simulink model "indicator_controller"  (R2025a)
settings: Solver=VariableStepAuto  StartTime=0.0  StopTime=10.0  RelTol=1e-3
settings Model: Creator=admin  LastModifiedBy=admin

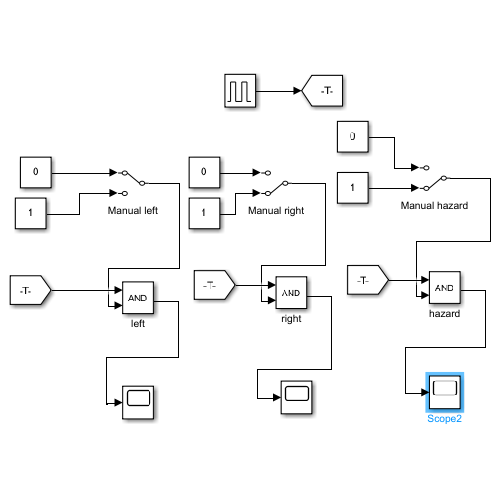
[thumbnail: Simulink's stored preview of the top-level diagram]
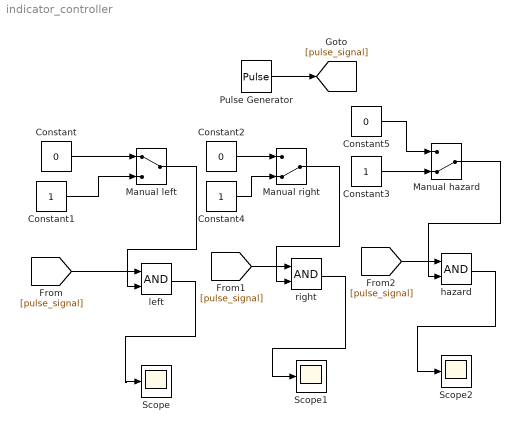
== system indicator_controller ==
  Constant : Constant  Value=0
  Constant1 : Constant
  Constant2 : Constant  Value=0
  Constant3 : Constant
  Constant4 : Constant
  Constant5 : Constant  Value=0
  Manual hazard : ManualSwitch  CurrentSetting=0
  Manual left : ManualSwitch
  Manual right : ManualSwitch  CurrentSetting=0
  Pulse Generator : DiscretePulseGenerator  PulseType=Time based  PulseWidth=50
  Scope : Scope
      settings: ActiveDisplayYMinimum=-1  ActiveDisplayYMaximum=1
  Scope1 : Scope
      settings: ActiveDisplayYMinimum=-0.12499999999999997  ActiveDisplayYMaximum=1.125
  Scope2 : Scope
      settings: ActiveDisplayYMinimum=-0.12499999999999997  ActiveDisplayYMaximum=1.125  DataLoggingVariableName=ScopeData2
  hazard : Logic  AllPortsSameDT=off  OutDataTypeStr=boolean
  left : Logic  AllPortsSameDT=off  OutDataTypeStr=boolean
  right : Logic  AllPortsSameDT=off  OutDataTypeStr=boolean
  wires:
  Manual left/1 -> left/2
  Manual right/1 -> right/2
  Manual hazard/1 -> hazard/2
  left/1 -> Scope/1
  right/1 -> Scope1/1
  hazard/1 -> Scope2/1
  Pulse Generator/1 -> [pulse_signal]
  [pulse_signal] -> left/1
  [pulse_signal] -> right/1
  [pulse_signal] -> hazard/1
  Constant/1 -> Manual left/1
  Constant1/1 -> Manual left/2
  Constant2/1 -> Manual right/1
  Constant4/1 -> Manual right/2
  Constant5/1 -> Manual hazard/1
  Constant3/1 -> Manual hazard/2
